simulink model "multisignal"  (R2018b)
settings: Solver=VariableStepAuto  StartTime=0.0  StopTime=10.0  RelTol=1e-3
settings Model: Creator=kekos  LastModifiedBy=kekos

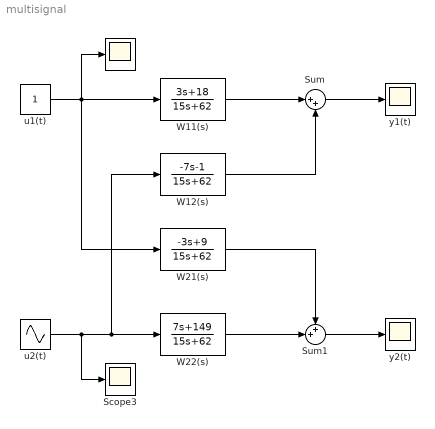
== system multisignal ==
  " " : Scope
  Scope3 : Scope
  Sum : Sum  Inputs=|++
  Sum1 : Sum  Inputs=++|
  W11(s) : TransferFcn  Numerator=[3 18]  Denominator=[15 62]
  W12(s) : TransferFcn  Numerator=[-7 -1]  Denominator=[15 62]
  W21(s) : TransferFcn  Numerator=[-3 9]  Denominator=[15 62]
  W22(s) : TransferFcn  Numerator=[7 149]  Denominator=[15 62]
  "u1(t) " : Constant
  u2(t) : Sin  Amplitude=2  SampleTime=0
  y1(t) : Scope
  y2(t) : Scope
  wires:
  u2(t)/1 -> Scope3/1, W12(s)/1, W22(s)/1
  "u1(t) "/1 -> " "/1, W11(s)/1, W21(s)/1
  W11(s)/1 -> Sum/1
  W12(s)/1 -> Sum/2
  W21(s)/1 -> Sum1/1
  W22(s)/1 -> Sum1/2
  Sum/1 -> y1(t)/1
  Sum1/1 -> y2(t)/1
